simulink subsystem "RMS"  (R2024b)
settings: Solver=VariableStepAuto  StartTime=0.0  StopTime=10.0  RelTol=1e-3
settings Model: Creator=Mohammed Hany  LastModifiedBy=Mohammed Hany

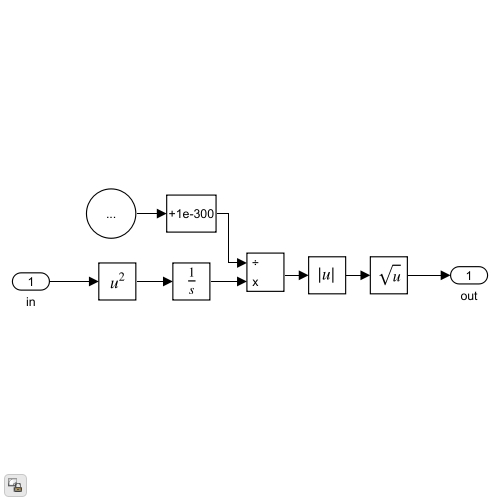
[thumbnail: Simulink's stored preview of the top-level diagram]
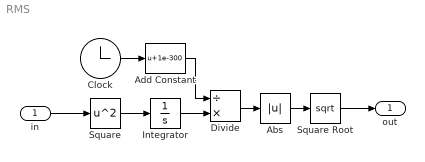
== system RMS ==
  in : Inport
  Abs : Abs  SaturateOnIntegerOverflow=off
  Add Constant : Bias  Bias=1e-300  SaturateOnIntegerOverflow=off
  Clock : Clock
  Divide : Product  Inputs=/*
  Integrator : Integrator
  Square : Math  Operator=square
  Square Root : Sqrt
  out : Outport
  wires:
  Divide/1 -> Abs/1
  Square Root/1 -> out/1
  in/1 -> Square/1
  Clock/1 -> Add Constant/1
  Integrator/1 -> Divide/2
  Add Constant/1 -> Divide/1
  Square/1 -> Integrator/1
  Abs/1 -> Square Root/1
